simulink model "bluetoothnxttest"  (R2014a)
settings: Solver=ode3  SolverMode=SingleTasking  StartTime=0.0  StopTime=inf  RelTol=1e-3
libraries: legonxtlib x2, simulink x1
settings Model: ExtModeTrigDuration=2  Creator=nrattner  LastModifiedBy=nrattner
settings OptimizationCC: OptimizeModelRefInitCode=on  LifeSpan=1
settings DebuggingCC: UnderspecifiedInitializationDetection=Classic  SolverPrmCheckMsg=none
settings HardwareCC: ProdLargestAtomicInteger=Long  ProdLargestAtomicFloat=Float  ProdEndianess=LittleEndian  ProdHWDeviceType=ARM Compatible->ARM 7
settings RTWCC: SystemTargetFile=realtime.tlc  GenerateMakefile=off  TemplateMakefile=realtime.tmf  Description=Run on Target Hardware  RTWVerbose=off  ProcessScript=realtime_make_rtw_hook
settings STFCustomTargetCC: TargetLibSuffix=.a  GenerateSampleERTMain=on  ConcurrentExecutionCompliant=off  GeneratePreprocessorConditionals=Use local settings  ERTCustomFileBanners=on  SupportNonInlinedSFcns=off  SupportVariableSizeSignals=on  MATLABClassNameForMDSCustomization=Simulink.SoftwareTarget.ERTCustomization  GRTInterface=off  SystemTargetFile=realtime.tlc
settings ERTTargetCC: CombineOutputUpdateFcns=off  SupportContinuousTime=on  SupportVariableSizeSignals=on  ExtModeTransport=2  ExtModeMexFile=ext_serial_win32_comm_no_acks_rtt  ExtModeMexArgs=0 1 9600  ERTSrcFileBannerTemplate=realtime_code_template.cgt  ERTHdrFileBannerTemplate=realtime_code_template.cgt  ERTDataSrcFileTemplate=realtime_code_template.cgt  ERTDataHdrFileTemplate=realtime_code_template.cgt  ERTCustomFileTemplate=realtime_file_process.tlc

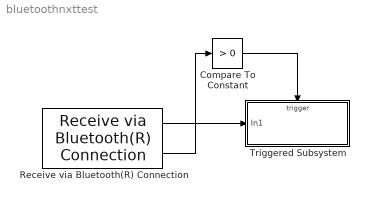
== system bluetoothnxttest ==
  Compare To Constant : simulink/Logic and Bit Operations/Compare To Constant  relop=>  const=0  OutDataTypeStr=boolean
  Receive via Bluetooth(R) Connection : legonxtlib/Receive via Bluetooth(R) Connection  mailbox=1  dataType=uint8  dataSize=1  sampleTime=0.1
  Triggered Subsystem : Subsystem  TreatAsAtomicUnit=on
  wires:
  Receive via Bluetooth(R) Connection/1 -> Triggered Subsystem/1(In1)
  Compare To Constant/1 -> Triggered Subsystem/Trigger
  Receive via Bluetooth(R) Connection/2 -> Compare To Constant/1

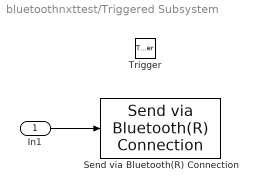
== system bluetoothnxttest/Triggered Subsystem ==
  In1 : Inport
  Trigger : TriggerPort
  Send via Bluetooth(R) Connection : legonxtlib/Send via Bluetooth(R) Connection  mailbox=1
  wires:
  In1/1 -> Send via Bluetooth(R) Connection/1
